simulink model "ROV_Simulator"  (R2023b)
settings: Solver=ode45  StartTime=0.0  StopTime=100  FixedStep=0.0001  MaxStep=0.0001  RelTol=1e-3
InitFcn:
  | init_params
  | 
  | vehicle_parameters_vita1_simu2vita
model workspace (MAT data in the model file):
  PID_params = [219.545279942 3.70519601588 93.8828385991 194.811835155 6.72701520051 121.59112254 154.922739587 1.92908191949 101.939011964 1.23491492885 1.15087256702 0.897835335235 0.858804638878 3.40602843271 0.73871001899 1.02484674583 4.65741084383 0.363408187927]
  PID_pitch = [0 0 0]
  PID_roll = [0 0 0]
  PID_x = [0 0 0]
  PID_y = [0 0 0]
  PID_yaw = [0.04 0 0.18]
  PID_z = [0 0 0]
values from neighbouring files (symbols this model uses):
  actuators_tconst = ones(qty_actuators, 1)*0.1754    [vehicle_parameters_vita1_simu2vita.m]
  Dlf = -[X_u;         Y_v;         Z_w;         K_p;         M_q;         N_r]    [vehicle_parameters_vita1_simu2vita.m]
  Dqf = -[X_u_u;         Y_v_v;         Z_w_w;         K_p_p;         M_q_q;         N_r_r]    [vehicle_parameters_vita1_simu2vita.m]
  I_b = diag([I_x; I_y; I_z])    [vehicle_parameters_vita1_simu2vita.m]
  init_vehicle_linear_vel = [0 0 0]'    [init_params.m]
  init_vehicle_position = [0 0 0]'    [init_params.m]
  last_waypoint_thresh = Parameters.reference.path.last_waypoint_thresh    [init_params.m]
  m = 25    [vehicle_parameters_vita1_simu2vita.m]
  Ma = -diag([X_u_dot; Y_v_dot; Z_w_dot; K_p_dot; M_q_dot; N_r_dot])    [vehicle_parameters_vita1_simu2vita.m]
  nlinear_sf = 400    [init_params.m]
  path_ref_mask = Parameters.reference.path.reference_mask    [init_params.m]
  pos_sample_freq = 4    [init_params.m]
  qty_actuators = 8    [vehicle_parameters_vita1_simu2vita.m]
  r_b = [0; 0; -0.08]    [vehicle_parameters_vita1_simu2vita.m]
  r_g = [0; 0; 0.02]    [vehicle_parameters_vita1_simu2vita.m]
  ref_switch = 1    [init_params.m]
  ref_waypoints = Parameters.reference.path.waypoints    [init_params.m]
  rho = 1028    [vehicle_parameters_vita1_simu2vita.m]
  step_signal = Parameters.reference.stage_step_signal    [init_params.m]
  thrust_inferior = ones(qty_actuators, 1)*(-39.91)    [vehicle_parameters_vita1_simu2vita.m]
  thrust_sup = ones(qty_actuators, 1)*51.48    [vehicle_parameters_vita1_simu2vita.m]
  thruster_effectiveness_matrix = thruster_effectiveness_matrix *                               thruster_effectiveness    [vehicle_parameters_vita1_simu2vita.m]
  vol = 0.02432    [vehicle_parameters_vita1_simu2vita.m]
  waypoint_thresh = Parameters.reference.path.waypoint_thresh    [init_params.m]
libraries: slpidlib x6, sharedutil x3, aerolibutil x3, sharedtransform x2, aerolibconvert2 x1, dspswit3 x1
(part 1 of 2)
settings Model: PacingRate=0.890000  Creator=spades  LastModifiedBy=HP
settings SolverCC: ConcurrentTasks=on  AlgebraicLoopSolver=TrustRegion  AutoInsertRateTranBlk=on
settings OptimizationCC: EnhancedBackFolding=on  PassReuseOutputArgsThreshold=0  MaxStackSize=64  OptimizeBlockOrder=speed  DifferentSizesBufferReuse=on
settings DebuggingCC: ReadBeforeWriteMsg=DisableAll  WriteAfterWriteMsg=DisableAll  WriteAfterReadMsg=DisableAll  InheritedTsInSrcMsg=none  ParameterTunabilityLossMsg=error  UnconnectedLineMsg=warning
settings HardwareCC: ProdBitPerLong=64  ProdHWDeviceType=Intel->x86-64 (Linux 64)
settings ModelReferenceCC: EnableRefExpFcnMdlSchedulingChecks=on
settings SFSimCC: MATLABDynamicMemAlloc=off
settings RTWCC: GenerateReport=on  Toolchain=Catkin  LaunchReport=on
settings CodeAppCC: ForceParamTrailComments=on  OperatorAnnotations=on
settings GRTTargetCC: TargetLangStandard=C89/C90 (ANSI)

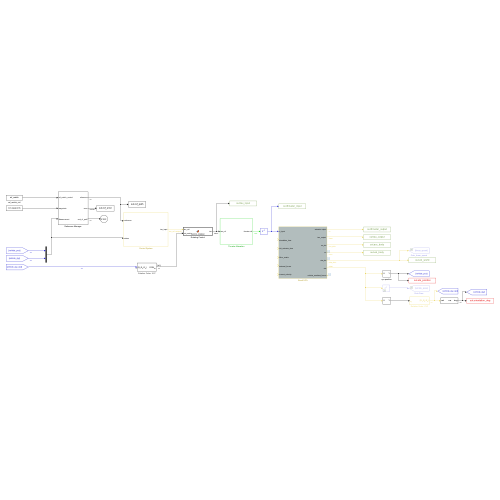
[thumbnail: Simulink's stored preview of the top-level diagram]
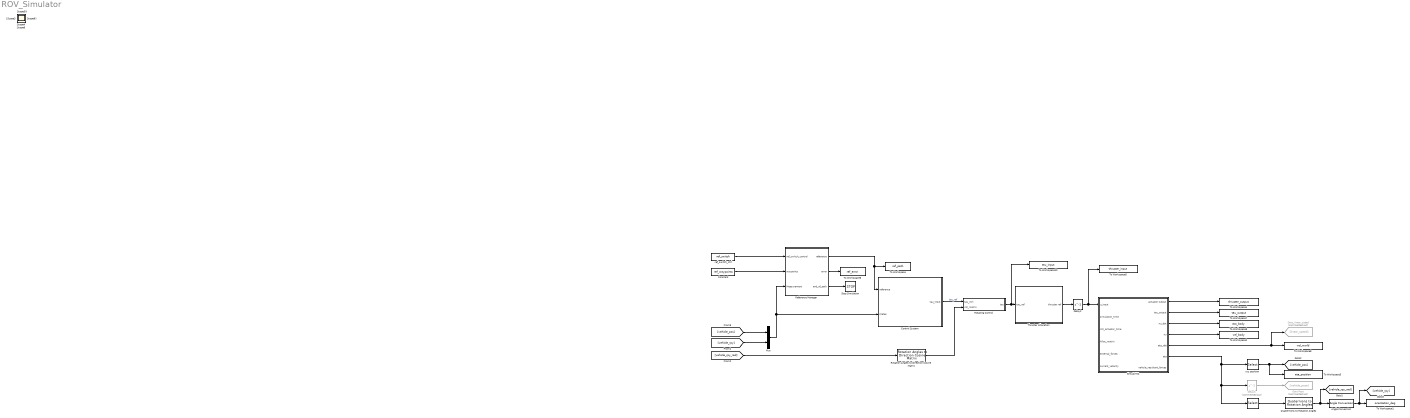
== system ROV_Simulator ==
  " " : Selector  InputPortWidth=7  IndexOptions=Index vector (dialog)  Indices=[4 5 6 7]  OutputSizes=1
  Angle Conversion : aerolibconvert2/Angle Conversion  IU=rad  OU=deg
  Constant : Constant  Value=ref_waypoints
  Control System : Subsystem
  Delay2 : Delay  DelayLength=1  InitialCondition=[0 0 0 0 0 0 0 0]'  SampleTime=1/nlinear_sf
  Delay3 : Delay  Commented=on  DelayLength=1  InitialCondition=[init_vehicle_position' init_vehicle_orientation']'  SampleTime=1/nlinear_sf
  Goto Pose : Goto  Commented=on  GotoTag=vehicle_pose
  Goto_linear_speed : Goto  Commented=on  GotoTag=linear_speed
  Mux : Mux  Inputs=2
  Quaternions to Rotation Angles : sharedtransform/Quaternions to Rotation Angles  rotationOrder=XYZ  aMode=aMode
  Reference Manager : Subsystem
  Rotating Control : MATLAB Function  TreatAsAtomicUnit=on
  Rotation Angles to Direction Cosine Matrix : sharedtransform/Rotation Angles to Direction Cosine Matrix  rotationOrder=XYZ  aMode=aMode
  Simu2VITA : Subsystem  mask{m_qty_actuators=qty_actuators, m_init_actuators_state=[0; 0; 0; 0; 0; 0; 0; 0], m_logic_op_use_custom_actuators_init_states=on, m_internal_init_actuators_time=0, m_logic_op_use_external_actuators_init_time=off, m_logic_op_use_external_time=off, m_thrust_sup=thrust_sup, m_thrust_inf=thrust_inferior, m_logic_op_thrust_saturation=on, m_actuators_tconst_vec=actuators_tconst, m_allocation_matrix=thruster_effectiveness_matrix, m_logic_op_external_alloc_mat=off, m_m=m, m_vol=vol, m_r_g=r_g, m_I_b=I_b, m_loigc_op_use_external_forces=off, m_Ma=Ma, m_Dlf_vec=Dlf, m_Dqf_vec=Dqf, m_current_velocity=[0.7 0 0]', m_loigc_op_use_external_current_velocity=off, m_g=9.81, m_rho=rho, m_r_b=r_b, m_eta_0=[init_vehicle_position' init_vehicle_orientation']', m_nu_0=[init_vehicle_linear_vel' init_vehicle_angular_vel']'}
      mask prompts: m_qty_actuators "Number of actuators on vehicle"; m_init_actuators_state "Actuators initial state values"; m_logic_op_use_custom_actuators_init_states "use custom initial state for actuators to start"; m_internal_init_actuators_time "Actuators initial time values"; m_logic_op_use_external_actuators_init_time "use custom initial time for actuators to start"; m_logic_op_use_external_time "use external clock reference"; m_thrust_sup "Thrust superior saturation limits"; m_thrust_inf "Thrust lower saturation limits"; m_logic_op_thrust_saturation "use thrust saturation"; m_actuators_tconst_vec "Time Constant values"; m_allocation_matrix "Allocation Matrix"; m_logic_op_external_alloc_mat "use external allocation matrix"; m_m "Vehicle Total Mass"; m_vol "Vehicle Total Volume"; m_r_g "Vehicle center of gravity w.r.t. vehicle control point"; m_I_b "Intertia Matrix"; m_loigc_op_use_external_forces "enable external forces and moments"; m_Ma "Addded Mass Matrix"; m_Dlf_vec "Drag Linear Factor"; m_Dqf_vec "Drag Non Linear Factor"; m_current_velocity "Fluid current velocity"; m_loigc_op_use_external_current_velocity "use external fluid current velocity"; m_g "Gravity Constant"; m_rho "Fluid Constant"; m_r_b "Vehicle center of bouyance w.r.t. vehicle body frame"; m_eta_0 "Initial pose of the vehicle -- [pos quat]'"; m_nu_0 "Initial velocity and gyros of the vehicle -- [u v w p q r]'"
      mask help: $ \eta = 0 $
      mask init:
      | assert((numel(m_qty_actuators) == 1 && m_qty_actuators >= 0), 'The number of actuators must be a non-negative   scalar.');
      | 
      | if(m_qty_actuators == 0)
      |    
      |     m_logic_op_external_alloc_mat = false;
      |     m_allocation_matrix = zeros(6,1);
      |     m_init_actuators_state = 0;
      |     m_internal_init_actuators_time = 0;
      |     m_actuators_tconst_vec = 1;
      |     m_thrust_sup = 0;
      |     m_thrust_inf = 0;
      |     m_logic_op_thrust_saturation = false;
      |     
      | else
      |     
      |     if(~m_logic_op_use_custom_actuators_init_states)
      |         m_init_actuators_state = zeros(m_qty_actuators,1);
      |     end
      |     
      |     if(~m_logic_op_use_external_actuators_init_time)
      |         m_internal_init_actuators_time = zeros(m_qty_actuators,1);
      |     end
      |     
      |     if(m_logic_op_thrust_saturation)
      |         assert(isequal(size(m_thrust_sup), [m_qty_actuators 1]));
      |         assert(isequal(size(m_thrust_inf), [m_qty_actuators 1]));
      |     end
      |     
      |     assert(isequal(size(m_init_actuators_state), [m_qty_actuators 1]), ...
      |         'Initial actuator state vector must be a column vector and agree with the number of actuators specified.');
      |     
      |     assert(isequal(size(m_internal_init_actuators_time), [m_qty_actuators 1]), ...
      |         'Initial actuator time vector must be a column vector and agree with the number of actuators specified.');
      |     
      | end
      | 
      | if(~m_logic_op_external_alloc_mat)
      | 
      |     assert(isequal(size(m_allocation_matrix), [6 numel(m_init_actuators_state)]));
      | 
      | end
      | 
      | assert(isequal(size(m_r_g), [3 1]), 'Center of gravity must be a 3x1 column vector.');
      | assert(isequal(size(m_r_b), [3 1]), 'Center of bouyancy must be a 3x1 column vector.');
      | assert(isequal(size(m_eta_0), [7 1]), 'Initial pose state w.r.t. NED must be a 7x1 column vector.');
      | assert(abs(norm(m_eta_0(4:7,1)) - 1) < 0.00001, 'Initial orientation state quaternion must have unitary norm.')
      | assert(isequal(size(m_nu_0), [6 1]), 'Initial velocity state w.r.t. body must be a 6x1 column vector.');
      | assert(isequal(size(m_I_b), [3 3]), 'Inertia matrix w.r.t. body must be a 3x3 matrix.');
      | assert(isequal(size(m_Ma), [6 6]), 'Added mass matrix must be a 6x6 matrix.');
      | assert(isequal(size(m_current_velocity), [3 1]), 'Current velocity must be a 3x1 column vector.');
      | assert(isequal(size(m_m), [1 1]), 'Mass must be a scalar.');
      | assert(isequal(size(m_vol), [1 1]), 'The volume of the vehicle must be a scalar.');
      | assert(isequal(size(m_g), [1 1]), 'Gravity must be a scalar.');
      | assert(isequal(size(m_rho), [1 1]), 'Fluid density must be a scalar.');
      | assert(isequal(size(m_Dlf_vec), [6 1]), 'Linear Drag Matrix is assumed to be diagonal and should be entered as a 6x1 vector.');
      | assert(isequal(size(m_Dqf_vec), [6 1]), 'Non-Linear Drag Matrix is assumed to be diagonal and should be entered as a 6x1 vector.');
      | 
      | m_W = m_m*m_g;
      | 
      | m_B = -m_vol*m_g*m_rho;
      | 
      | m_Smtrx_r_g = [0 -m_r_g(3) m_r_g(2); ... 
      |              m_r_g(3) 0 -m_r_g(1); ... 
      |             -m_r_g(2) m_r_g(1) 0];  
      | 
      | m_M = [m_m*eye(3) -m_m*m_Smtrx_r_g; ...
      |      m_m*m_Smtrx_r_g m_I_b];
      | 
      | m_Dlf = diag(m_Dlf_vec);
      | m_Dqf = diag(m_Dqf_vec);
      | 
      | m_Ad = diag((-1./m_actuators_tconst_vec));
      | m_Bd = -m_Ad;
      | m_Cd = diag(ones(size(m_Ad, 2), 1));
      | m_Dd = zeros(numel(m_actuators_tconst_vec), numel(m_actuators_tconst_vec));
      mask Callback m_logic_op_use_custom_actuators_init_states:
      | p = Simulink.Mask.get(gcb);
      | a = p.Parameters(2);
      | 
      | cur_param_val_on = ...
      |     (strcmp(get_param(gcb, 'm_logic_op_use_custom_actuators_init_states'), 'on') ~= 0);
      | 
      | if (cur_param_val_on)
      | 
      |     for i = 1
      |         a(i).set('Enabled', 'on');
      |     end
      | 
      | else
      | 
      |     for i = 1
      |         a(i).set('Enabled', 'off');
      |     end
      | 
      | end
      mask Callback m_logic_op_use_external_actuators_init_time:
      | p = Simulink.Mask.get(gcb);
      | a = p.Parameters(4);
      | 
      | cur_param_val_on = ...
      |     (strcmp(get_param(gcb, 'm_logic_op_use_external_actuators_init_time'), 'on') ~= 0);
      | 
      | if (cur_param_val_on)
      | 
      |     for i = 1
      |         a(i).set('Enabled', 'on');
      |     end
      | 
      | else
      | 
      |     for i = 1
      |         a(i).set('Enabled', 'off');
      |     end
      | 
      | end
      mask Callback m_logic_op_thrust_saturation:
      | p = Simulink.Mask.get(gcb);
      | a = p.Parameters(7:8);
      | 
      | cur_param_val_on = ...
      |     (strcmp(get_param(gcb, 'm_logic_op_thrust_saturation'), 'on') ~= 0);
      | 
      | if (cur_param_val_on)
      | 
      |     for i = 1:2
      |         a(i).set('Enabled', 'on');
      |     end
      | 
      | else
      | 
      |     for i = 1:2
      |         a(i).set('Enabled', 'off');
      |     end
      | 
      | end
      mask Callback m_logic_op_external_alloc_mat:
      | p = Simulink.Mask.get(gcb);
      | a = p.Parameters(11);
      | 
      | cur_param_val_on = ...
      |     (strcmp(get_param(gcb, 'm_logic_op_external_alloc_mat'), 'on') ~= 0);
      | 
      | if (cur_param_val_on)
      | 
      |     for i = 1
      |         a(i).set('Enabled', 'off');
      |     end
      | 
      | else
      | 
      |     for i = 1
      |         a(i).set('Enabled', 'on');
      |     end
      | 
      | end
      mask Callback m_loigc_op_use_external_current_velocity:
      | p = Simulink.Mask.get(gcb);
      | a = p.Parameters(21);
      | 
      | cur_param_val_on = ...
      |     (strcmp(get_param(gcb, 'm_loigc_op_use_external_current_velocity'), 'on') ~= 0);
      | 
      | if (cur_param_val_on)
      | 
      |     for i = 1
      |         a(i).set('Enabled', 'off');
      |     end
      | 
      | else
      | 
      |     for i = 1
      |         a(i).set('Enabled', 'on');
      |     end
      | 
      | end
      mask DialogControl act_system Prompt: Actuator Module
      mask DialogControl act_start_group Prompt: Start options
      mask DialogControl thrust_sat_options Prompt: Thrust saturation options
      mask DialogControl act_evo_group Prompt: Evolution options
      mask DialogControl vehicle_input_tab Prompt: Allocation Module
      mask DialogControl vehicle_dynamic_tab Prompt: Vehicle Dynamic Parameters
      mask DialogControl rigid_body_comp Prompt: Rigid-body Components
      mask DialogControl m_vol Tooltip: Liters
      mask DialogControl hydro_dynam_comp Prompt: Hydrodanymic Components
      mask DialogControl hydro_static_comp Prompt: Hydrostatic Components
      mask DialogControl init_state Prompt: Initial state of the vehicle
      mask DialogControl m_eta_0 Tooltip: Pose state of the vehicle [pose quat]', with pose in meters w.r.t. NED
  Stop Simulation : Stop
  Thruster Allocation : Subsystem
  To Workspace : ToWorkspace  VariableName=ref_path  SaveFormat=Timeseries  SampleTime=-1
  To Workspace1 : ToWorkspace  VariableName=orientation_deg  SaveFormat=Timeseries  SampleTime=-1
  To Workspace10 : ToWorkspace  VariableName=tau_input  SaveFormat=Timeseries  SampleTime=-1
  To Workspace2 : ToWorkspace  VariableName=vel_body  SaveFormat=Timeseries  SampleTime=1/pos_sample_freq
  To Workspace3 : ToWorkspace  VariableName=eta_position  SaveFormat=Timeseries  SampleTime=-1
  To Workspace4 : ToWorkspace  VariableName=thruster_output  SaveFormat=Timeseries  SampleTime=-1
  To Workspace5 : ToWorkspace  VariableName=thruster_input  SaveFormat=Timeseries  SampleTime=-1
  To Workspace6 : ToWorkspace  VariableName=ref_error  SaveFormat=Timeseries  SampleTime=-1
  To Workspace7 : ToWorkspace  VariableName=tau_output  SaveFormat=Timeseries  SampleTime=-1
  To Workspace8 : ToWorkspace  VariableName=vel_world  SaveFormat=Timeseries  SampleTime=1/pos_sample_freq
  To Workspace9 : ToWorkspace  VariableName=acc_body  SaveFormat=Timeseries  SampleTime=1/pos_sample_freq
  ref_switch_ctrl : Constant  Value=ref_switch
  xyz position : Selector  InputPortWidth=7  IndexOptions=Index vector (dialog)  Indices=[1 2 3]  OutputSizes=1
  Scope{,1..6,9..10,13..15,18..19} (14 alike) : Scope
  wires:
  Simu2VITA/6(eta) -> " "/1, Delay3/1, xyz position/1
  Delay3/1 -> Goto Pose/1
  Simu2VITA/4(nu) -> To Workspace2/1
  xyz position/1 -> [vehicle_pos], To Workspace3/1
  " "/1 -> Quaternions to Rotation Angles/1
  Quaternions to Rotation Angles/1 -> Angle Conversion/1, [vehicle_rpy_rad]
  Simu2VITA/1(actuator output) -> To Workspace4/1
  Simu2VITA/5(eta_dot) -> To Workspace8/1, Goto_linear_speed/1
  [vehicle_pos] -> Mux/1
  Mux/1 -> Reference Manager/3(Measurement), Control System/2(states)
  [vehicle_rpy] -> Mux/2
  Simu2VITA/2("tau_output ") -> To Workspace7/1
  Simu2VITA/3(nu_dot) -> To Workspace9/1
  Thruster Allocation/1(thruster ref) -> Delay2/1
  Delay2/1 -> To Workspace5/1, Simu2VITA/1(u_input)
  Rotation Angles to Direction Cosine Matrix/1 -> Rotating Control/2(rot_matrix)
  [vehicle_rpy_rad] -> Rotation Angles to Direction Cosine Matrix/1
  Control System/1(tau_input) -> Rotating Control/1(tau_ctrl)  "tau_ref"
  Angle Conversion/1 -> [vehicle_rpy], To Workspace1/1
  Rotating Control/1(tau) -> To Workspace10/1, Thruster Allocation/1(tau_ref)
  Reference Manager/1(reference) -> To Workspace/1, Control System/1(reference)
  Reference Manager/2(error) -> To Workspace6/1
  ref_switch_ctrl/1 -> Reference Manager/1(ref_switch_control)
  Constant/1 -> Reference Manager/2(waypoints)
  Reference Manager/3(end_of_path) -> Stop Simulation/1

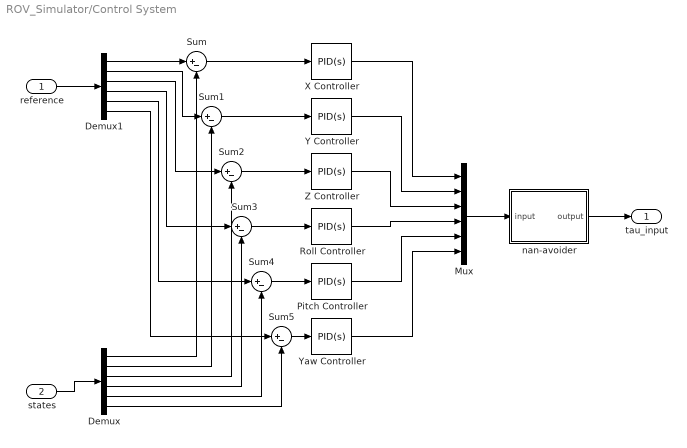
== system ROV_Simulator/Control System ==
  reference : Inport
  states : Inport  Port=2
  Demux : Demux  Outputs=6
  Demux1 : Demux  Outputs=6
  Mux : Mux  Inputs=6
  Pitch Controller : slpidlib/PID Controller  Controller=PID  Form=Parallel  TimeDomain=Continuous-time  UseExternalTs=off  SampleTime=-1  IntegratorMethod=Forward Euler  FilterMethod=Forward Euler  ControllerParametersSource=internal  P=PID_params(13)  I=PID_params(14)  UseKiTs=off  D=PID_params(15)  N=100  UseFilter=on  TunerSelectOption=Transfer Function Based (PID Tuner App)  InitialConditionSource=internal  InitialConditionForIntegrator=0  InitialConditionForFilter=0  DifferentiatorICPrevScaledInput=0  ExternalReset=none  TrackingMode=off  Kt=1  LimitOutput=off  SatLimitsSource=internal  UpperSaturationLimit=inf  LowerSaturationLimit=-inf  LinearizeAsGain=on  AntiWindupMode=none  Kb=1  LimitIntegrator=off  UpperIntegratorSaturationLimit=inf  LowerIntegratorSaturationLimit=-inf  POutMin=[]  POutMax=[]  IOutMin=[]  IOutMax=[]  DOutMin=[]  DOutMax=[]  NOutMin=[]  NOutMax=[]  SumOutMin=[]  SumOutMax=[]  SaturationOutMin=[]  SaturationOutMax=[]  PParamMin=[]  PParamMax=[]  IParamMin=[]  IParamMax=[]  DParamMin=[]  DParamMax=[]  NParamMin=[]  NParamMax=[]  KbParamMin=[]  KbParamMax=[]  KtParamMin=[]  KtParamMax=[]  KbOutMin=[]  KbOutMax=[]  KtOutMin=[]  KtOutMax=[]  IntegratorOutMin=[]  IntegratorOutMax=[]  FilterOutMin=[]  FilterOutMax=[]  SumI1OutMin=[]  SumI1OutMax=[]  SumI2OutMin=[]  SumI2OutMax=[]  SumI3OutMin=[]  SumI3OutMax=[]  SumI4OutMin=[]  SumI4OutMax=[]  SumDOutMin=[]  SumDOutMax=[]  DifferentiatorOutMin=[]  DifferentiatorOutMax=[]  FilterDiffOutCoefMin=[]  FilterDiffOutCoefMax=[]  ReciprocalOutMin=[]  ReciprocalOutMax=[]  SumDenOutMin=[]  SumDenOutMax=[]  SumNumOutMin=[]  SumNumOutMax=[]  DivideOutMin=[]  DivideOutMax=[]  UdiffTsProdOutMin=[]  UdiffTsProdOutMax=[]  NTsProdOutMin=[]  NTsProdOutMax=[]  UintegralTsProdOutMin=[]  UintegralTsProdOutMax=[]  UngainTsProdOutMin=[]  UngainTsProdOutMax=[]  ClampingZeroOutDataTypeStr=Inherit: Inherit via back propagation  ClampingZeroOutMin=[]  ClampingZeroOutMax=[]  FilterDenConstantOutDataTypeStr=Inherit: Inherit via back propagation  FilterDenConstantOutMin=[]  FilterDenConstantOutMax=[]  PCopyOutDataTypeStr=Inherit: Inherit via back propagation  PCopyOutMin=[]  PCopyOutMax=[]  NCopyOutDataTypeStr=Inherit: Inherit via back propagation  NCopyOutMin=[]  NCopyOutMax=[]  IntegratorContinuousStateAttributes=''  IntegratorStateMustResolveToSignalObject=off  IntegratorRTWStateStorageClass=Auto  FilterContinuousStateAttributes=''  FilterStateMustResolveToSignalObject=off  FilterRTWStateStorageClass=Auto  ParallelPVariant=InternalParameters  IdealPVariant=Disabled  IVariant=InternalParameters  DVariant=InternalParameters  IntegratorVariant=Continuous  SatVariant=Disabled  AWVariant=Passthrough  PCopyVariant=Disabled  TRVariant=Disabled  FdbkBlocksVariant=Forward  IdealPFdbkVariant=Disabled  SatFdbkVariant=Disabled  DerivativeFilterVariant=ContFilter  NVariant=InternalParameters  NCopyVariant=Disabled  FilterICVariant=InternalICsFilter  IntegratorICVariant=InternalICs  ExternalResetVariant=Disabled  TRSumVariant=Passthrough  SumFdbkVariant=Disabled  SumVariant=Sum_PID  TsampFilterVariant=InternalTs  TsampNgainVariant=Passthrough  TsampIntegralVariant=Disabled_SignalSpec  ExternalSaturationOutDataTypeStr=Inherit: Same as second input
  Roll Controller : slpidlib/PID Controller  Controller=PID  Form=Parallel  TimeDomain=Continuous-time  UseExternalTs=off  SampleTime=-1  IntegratorMethod=Forward Euler  FilterMethod=Forward Euler  ControllerParametersSource=internal  P=PID_params(10)  I=PID_params(11)  UseKiTs=off  D=PID_params(12)  N=100  UseFilter=on  TunerSelectOption=Transfer Function Based (PID Tuner App)  InitialConditionSource=internal  InitialConditionForIntegrator=0  InitialConditionForFilter=0  DifferentiatorICPrevScaledInput=0  ExternalReset=none  TrackingMode=off  Kt=1  LimitOutput=off  SatLimitsSource=internal  UpperSaturationLimit=inf  LowerSaturationLimit=-inf  LinearizeAsGain=on  AntiWindupMode=none  Kb=1  LimitIntegrator=off  UpperIntegratorSaturationLimit=inf  LowerIntegratorSaturationLimit=-inf  POutMin=[]  POutMax=[]  IOutMin=[]  IOutMax=[]  DOutMin=[]  DOutMax=[]  NOutMin=[]  NOutMax=[]  SumOutMin=[]  SumOutMax=[]  SaturationOutMin=[]  SaturationOutMax=[]  PParamMin=[]  PParamMax=[]  IParamMin=[]  IParamMax=[]  DParamMin=[]  DParamMax=[]  NParamMin=[]  NParamMax=[]  KbParamMin=[]  KbParamMax=[]  KtParamMin=[]  KtParamMax=[]  KbOutMin=[]  KbOutMax=[]  KtOutMin=[]  KtOutMax=[]  IntegratorOutMin=[]  IntegratorOutMax=[]  FilterOutMin=[]  FilterOutMax=[]  SumI1OutMin=[]  SumI1OutMax=[]  SumI2OutMin=[]  SumI2OutMax=[]  SumI3OutMin=[]  SumI3OutMax=[]  SumI4OutMin=[]  SumI4OutMax=[]  SumDOutMin=[]  SumDOutMax=[]  DifferentiatorOutMin=[]  DifferentiatorOutMax=[]  FilterDiffOutCoefMin=[]  FilterDiffOutCoefMax=[]  ReciprocalOutMin=[]  ReciprocalOutMax=[]  SumDenOutMin=[]  SumDenOutMax=[]  SumNumOutMin=[]  SumNumOutMax=[]  DivideOutMin=[]  DivideOutMax=[]  UdiffTsProdOutMin=[]  UdiffTsProdOutMax=[]  NTsProdOutMin=[]  NTsProdOutMax=[]  UintegralTsProdOutMin=[]  UintegralTsProdOutMax=[]  UngainTsProdOutMin=[]  UngainTsProdOutMax=[]  ClampingZeroOutDataTypeStr=Inherit: Inherit via back propagation  ClampingZeroOutMin=[]  ClampingZeroOutMax=[]  FilterDenConstantOutDataTypeStr=Inherit: Inherit via back propagation  FilterDenConstantOutMin=[]  FilterDenConstantOutMax=[]  PCopyOutDataTypeStr=Inherit: Inherit via back propagation  PCopyOutMin=[]  PCopyOutMax=[]  NCopyOutDataTypeStr=Inherit: Inherit via back propagation  NCopyOutMin=[]  NCopyOutMax=[]  IntegratorContinuousStateAttributes=''  IntegratorStateMustResolveToSignalObject=off  IntegratorRTWStateStorageClass=Auto  FilterContinuousStateAttributes=''  FilterStateMustResolveToSignalObject=off  FilterRTWStateStorageClass=Auto  ParallelPVariant=InternalParameters  IdealPVariant=Disabled  IVariant=InternalParameters  DVariant=InternalParameters  IntegratorVariant=Continuous  SatVariant=Disabled  AWVariant=Passthrough  PCopyVariant=Disabled  TRVariant=Disabled  FdbkBlocksVariant=Forward  IdealPFdbkVariant=Disabled  SatFdbkVariant=Disabled  DerivativeFilterVariant=ContFilter  NVariant=InternalParameters  NCopyVariant=Disabled  FilterICVariant=InternalICsFilter  IntegratorICVariant=InternalICs  ExternalResetVariant=Disabled  TRSumVariant=Passthrough  SumFdbkVariant=Disabled  SumVariant=Sum_PID  TsampFilterVariant=InternalTs  TsampNgainVariant=Passthrough  TsampIntegralVariant=Disabled_SignalSpec  ExternalSaturationOutDataTypeStr=Inherit: Same as second input
  Sum{,1..5} (6 alike) : Sum  Inputs=|+-
  X Controller : slpidlib/PID Controller  Controller=PID  Form=Parallel  TimeDomain=Continuous-time  UseExternalTs=off  SampleTime=-1  IntegratorMethod=Forward Euler  FilterMethod=Forward Euler  ControllerParametersSource=internal  P=PID_params(1)  I=PID_params(2)  UseKiTs=off  D=PID_params(3)  N=100  UseFilter=on  TunerSelectOption=Transfer Function Based (PID Tuner App)  InitialConditionSource=internal  InitialConditionForIntegrator=0  InitialConditionForFilter=0  DifferentiatorICPrevScaledInput=0  ExternalReset=none  TrackingMode=off  Kt=1  LimitOutput=off  SatLimitsSource=internal  UpperSaturationLimit=inf  LowerSaturationLimit=-inf  LinearizeAsGain=on  AntiWindupMode=none  Kb=1  LimitIntegrator=off  UpperIntegratorSaturationLimit=inf  LowerIntegratorSaturationLimit=-inf  POutMin=[]  POutMax=[]  IOutMin=[]  IOutMax=[]  DOutMin=[]  DOutMax=[]  NOutMin=[]  NOutMax=[]  SumOutMin=[]  SumOutMax=[]  SaturationOutMin=[]  SaturationOutMax=[]  PParamMin=[]  PParamMax=[]  IParamMin=[]  IParamMax=[]  DParamMin=[]  DParamMax=[]  NParamMin=[]  NParamMax=[]  KbParamMin=[]  KbParamMax=[]  KtParamMin=[]  KtParamMax=[]  KbOutMin=[]  KbOutMax=[]  KtOutMin=[]  KtOutMax=[]  IntegratorOutMin=[]  IntegratorOutMax=[]  FilterOutMin=[]  FilterOutMax=[]  SumI1OutMin=[]  SumI1OutMax=[]  SumI2OutMin=[]  SumI2OutMax=[]  SumI3OutMin=[]  SumI3OutMax=[]  SumI4OutMin=[]  SumI4OutMax=[]  SumDOutMin=[]  SumDOutMax=[]  DifferentiatorOutMin=[]  DifferentiatorOutMax=[]  FilterDiffOutCoefMin=[]  FilterDiffOutCoefMax=[]  ReciprocalOutMin=[]  ReciprocalOutMax=[]  SumDenOutMin=[]  SumDenOutMax=[]  SumNumOutMin=[]  SumNumOutMax=[]  DivideOutMin=[]  DivideOutMax=[]  UdiffTsProdOutMin=[]  UdiffTsProdOutMax=[]  NTsProdOutMin=[]  NTsProdOutMax=[]  UintegralTsProdOutMin=[]  UintegralTsProdOutMax=[]  UngainTsProdOutMin=[]  UngainTsProdOutMax=[]  ClampingZeroOutDataTypeStr=Inherit: Inherit via back propagation  ClampingZeroOutMin=[]  ClampingZeroOutMax=[]  FilterDenConstantOutDataTypeStr=Inherit: Inherit via back propagation  FilterDenConstantOutMin=[]  FilterDenConstantOutMax=[]  PCopyOutDataTypeStr=Inherit: Inherit via back propagation  PCopyOutMin=[]  PCopyOutMax=[]  NCopyOutDataTypeStr=Inherit: Inherit via back propagation  NCopyOutMin=[]  NCopyOutMax=[]  IntegratorContinuousStateAttributes=''  IntegratorStateMustResolveToSignalObject=off  IntegratorRTWStateStorageClass=Auto  FilterContinuousStateAttributes=''  FilterStateMustResolveToSignalObject=off  FilterRTWStateStorageClass=Auto  ParallelPVariant=InternalParameters  IdealPVariant=Disabled  IVariant=InternalParameters  DVariant=InternalParameters  IntegratorVariant=Continuous  SatVariant=Disabled  AWVariant=Passthrough  PCopyVariant=Disabled  TRVariant=Disabled  FdbkBlocksVariant=Forward  IdealPFdbkVariant=Disabled  SatFdbkVariant=Disabled  DerivativeFilterVariant=ContFilter  NVariant=InternalParameters  NCopyVariant=Disabled  FilterICVariant=InternalICsFilter  IntegratorICVariant=InternalICs  ExternalResetVariant=Disabled  TRSumVariant=Passthrough  SumFdbkVariant=Disabled  SumVariant=Sum_PID  TsampFilterVariant=InternalTs  TsampNgainVariant=Passthrough  TsampIntegralVariant=Disabled_SignalSpec  ExternalSaturationOutDataTypeStr=Inherit: Same as second input
  Y Controller : slpidlib/PID Controller  Controller=PID  Form=Parallel  TimeDomain=Continuous-time  UseExternalTs=off  SampleTime=-1  IntegratorMethod=Forward Euler  FilterMethod=Forward Euler  ControllerParametersSource=internal  P=PID_params(4)  I=PID_params(5)  UseKiTs=off  D=PID_params(6)  N=100  UseFilter=on  TunerSelectOption=Transfer Function Based (PID Tuner App)  InitialConditionSource=internal  InitialConditionForIntegrator=0  InitialConditionForFilter=0  DifferentiatorICPrevScaledInput=0  ExternalReset=none  TrackingMode=off  Kt=1  LimitOutput=off  SatLimitsSource=internal  UpperSaturationLimit=inf  LowerSaturationLimit=-inf  LinearizeAsGain=on  AntiWindupMode=none  Kb=1  LimitIntegrator=off  UpperIntegratorSaturationLimit=inf  LowerIntegratorSaturationLimit=-inf  POutMin=[]  POutMax=[]  IOutMin=[]  IOutMax=[]  DOutMin=[]  DOutMax=[]  NOutMin=[]  NOutMax=[]  SumOutMin=[]  SumOutMax=[]  SaturationOutMin=[]  SaturationOutMax=[]  PParamMin=[]  PParamMax=[]  IParamMin=[]  IParamMax=[]  DParamMin=[]  DParamMax=[]  NParamMin=[]  NParamMax=[]  KbParamMin=[]  KbParamMax=[]  KtParamMin=[]  KtParamMax=[]  KbOutMin=[]  KbOutMax=[]  KtOutMin=[]  KtOutMax=[]  IntegratorOutMin=[]  IntegratorOutMax=[]  FilterOutMin=[]  FilterOutMax=[]  SumI1OutMin=[]  SumI1OutMax=[]  SumI2OutMin=[]  SumI2OutMax=[]  SumI3OutMin=[]  SumI3OutMax=[]  SumI4OutMin=[]  SumI4OutMax=[]  SumDOutMin=[]  SumDOutMax=[]  DifferentiatorOutMin=[]  DifferentiatorOutMax=[]  FilterDiffOutCoefMin=[]  FilterDiffOutCoefMax=[]  ReciprocalOutMin=[]  ReciprocalOutMax=[]  SumDenOutMin=[]  SumDenOutMax=[]  SumNumOutMin=[]  SumNumOutMax=[]  DivideOutMin=[]  DivideOutMax=[]  UdiffTsProdOutMin=[]  UdiffTsProdOutMax=[]  NTsProdOutMin=[]  NTsProdOutMax=[]  UintegralTsProdOutMin=[]  UintegralTsProdOutMax=[]  UngainTsProdOutMin=[]  UngainTsProdOutMax=[]  ClampingZeroOutDataTypeStr=Inherit: Inherit via back propagation  ClampingZeroOutMin=[]  ClampingZeroOutMax=[]  FilterDenConstantOutDataTypeStr=Inherit: Inherit via back propagation  FilterDenConstantOutMin=[]  FilterDenConstantOutMax=[]  PCopyOutDataTypeStr=Inherit: Inherit via back propagation  PCopyOutMin=[]  PCopyOutMax=[]  NCopyOutDataTypeStr=Inherit: Inherit via back propagation  NCopyOutMin=[]  NCopyOutMax=[]  IntegratorContinuousStateAttributes=''  IntegratorStateMustResolveToSignalObject=off  IntegratorRTWStateStorageClass=Auto  FilterContinuousStateAttributes=''  FilterStateMustResolveToSignalObject=off  FilterRTWStateStorageClass=Auto  ParallelPVariant=InternalParameters  IdealPVariant=Disabled  IVariant=InternalParameters  DVariant=InternalParameters  IntegratorVariant=Continuous  SatVariant=Disabled  AWVariant=Passthrough  PCopyVariant=Disabled  TRVariant=Disabled  FdbkBlocksVariant=Forward  IdealPFdbkVariant=Disabled  SatFdbkVariant=Disabled  DerivativeFilterVariant=ContFilter  NVariant=InternalParameters  NCopyVariant=Disabled  FilterICVariant=InternalICsFilter  IntegratorICVariant=InternalICs  ExternalResetVariant=Disabled  TRSumVariant=Passthrough  SumFdbkVariant=Disabled  SumVariant=Sum_PID  TsampFilterVariant=InternalTs  TsampNgainVariant=Passthrough  TsampIntegralVariant=Disabled_SignalSpec  ExternalSaturationOutDataTypeStr=Inherit: Same as second input
  Yaw Controller : slpidlib/PID Controller  Controller=PID  Form=Parallel  TimeDomain=Continuous-time  UseExternalTs=off  SampleTime=-1  IntegratorMethod=Forward Euler  FilterMethod=Forward Euler  ControllerParametersSource=internal  P=PID_params(16)  I=PID_params(17)  UseKiTs=off  D=PID_params(18)  N=100  UseFilter=on  TunerSelectOption=Transfer Function Based (PID Tuner App)  InitialConditionSource=internal  InitialConditionForIntegrator=0  InitialConditionForFilter=0  DifferentiatorICPrevScaledInput=0  ExternalReset=none  TrackingMode=off  Kt=1  LimitOutput=off  SatLimitsSource=internal  UpperSaturationLimit=inf  LowerSaturationLimit=-inf  LinearizeAsGain=on  AntiWindupMode=none  Kb=1  LimitIntegrator=off  UpperIntegratorSaturationLimit=inf  LowerIntegratorSaturationLimit=-inf  POutMin=[]  POutMax=[]  IOutMin=[]  IOutMax=[]  DOutMin=[]  DOutMax=[]  NOutMin=[]  NOutMax=[]  SumOutMin=[]  SumOutMax=[]  SaturationOutMin=[]  SaturationOutMax=[]  PParamMin=[]  PParamMax=[]  IParamMin=[]  IParamMax=[]  DParamMin=[]  DParamMax=[]  NParamMin=[]  NParamMax=[]  KbParamMin=[]  KbParamMax=[]  KtParamMin=[]  KtParamMax=[]  KbOutMin=[]  KbOutMax=[]  KtOutMin=[]  KtOutMax=[]  IntegratorOutMin=[]  IntegratorOutMax=[]  FilterOutMin=[]  FilterOutMax=[]  SumI1OutMin=[]  SumI1OutMax=[]  SumI2OutMin=[]  SumI2OutMax=[]  SumI3OutMin=[]  SumI3OutMax=[]  SumI4OutMin=[]  SumI4OutMax=[]  SumDOutMin=[]  SumDOutMax=[]  DifferentiatorOutMin=[]  DifferentiatorOutMax=[]  FilterDiffOutCoefMin=[]  FilterDiffOutCoefMax=[]  ReciprocalOutMin=[]  ReciprocalOutMax=[]  SumDenOutMin=[]  SumDenOutMax=[]  SumNumOutMin=[]  SumNumOutMax=[]  DivideOutMin=[]  DivideOutMax=[]  UdiffTsProdOutMin=[]  UdiffTsProdOutMax=[]  NTsProdOutMin=[]  NTsProdOutMax=[]  UintegralTsProdOutMin=[]  UintegralTsProdOutMax=[]  UngainTsProdOutMin=[]  UngainTsProdOutMax=[]  ClampingZeroOutDataTypeStr=Inherit: Inherit via back propagation  ClampingZeroOutMin=[]  ClampingZeroOutMax=[]  FilterDenConstantOutDataTypeStr=Inherit: Inherit via back propagation  FilterDenConstantOutMin=[]  FilterDenConstantOutMax=[]  PCopyOutDataTypeStr=Inherit: Inherit via back propagation  PCopyOutMin=[]  PCopyOutMax=[]  NCopyOutDataTypeStr=Inherit: Inherit via back propagation  NCopyOutMin=[]  NCopyOutMax=[]  IntegratorContinuousStateAttributes=''  IntegratorStateMustResolveToSignalObject=off  IntegratorRTWStateStorageClass=Auto  FilterContinuousStateAttributes=''  FilterStateMustResolveToSignalObject=off  FilterRTWStateStorageClass=Auto  ParallelPVariant=InternalParameters  IdealPVariant=Disabled  IVariant=InternalParameters  DVariant=InternalParameters  IntegratorVariant=Continuous  SatVariant=Disabled  AWVariant=Passthrough  PCopyVariant=Disabled  TRVariant=Disabled  FdbkBlocksVariant=Forward  IdealPFdbkVariant=Disabled  SatFdbkVariant=Disabled  DerivativeFilterVariant=ContFilter  NVariant=InternalParameters  NCopyVariant=Disabled  FilterICVariant=InternalICsFilter  IntegratorICVariant=InternalICs  ExternalResetVariant=Disabled  TRSumVariant=Passthrough  SumFdbkVariant=Disabled  SumVariant=Sum_PID  TsampFilterVariant=InternalTs  TsampNgainVariant=Passthrough  TsampIntegralVariant=Disabled_SignalSpec  ExternalSaturationOutDataTypeStr=Inherit: Same as second input
  Z Controller : slpidlib/PID Controller  Controller=PID  Form=Parallel  TimeDomain=Continuous-time  UseExternalTs=off  SampleTime=-1  IntegratorMethod=Forward Euler  FilterMethod=Forward Euler  ControllerParametersSource=internal  P=PID_params(7)  I=PID_params(8)  UseKiTs=off  D=PID_params(9)  N=100  UseFilter=on  TunerSelectOption=Transfer Function Based (PID Tuner App)  InitialConditionSource=internal  InitialConditionForIntegrator=0  InitialConditionForFilter=0  DifferentiatorICPrevScaledInput=0  ExternalReset=none  TrackingMode=off  Kt=1  LimitOutput=off  SatLimitsSource=internal  UpperSaturationLimit=inf  LowerSaturationLimit=-inf  LinearizeAsGain=on  AntiWindupMode=none  Kb=1  LimitIntegrator=off  UpperIntegratorSaturationLimit=inf  LowerIntegratorSaturationLimit=-inf  POutMin=[]  POutMax=[]  IOutMin=[]  IOutMax=[]  DOutMin=[]  DOutMax=[]  NOutMin=[]  NOutMax=[]  SumOutMin=[]  SumOutMax=[]  SaturationOutMin=[]  SaturationOutMax=[]  PParamMin=[]  PParamMax=[]  IParamMin=[]  IParamMax=[]  DParamMin=[]  DParamMax=[]  NParamMin=[]  NParamMax=[]  KbParamMin=[]  KbParamMax=[]  KtParamMin=[]  KtParamMax=[]  KbOutMin=[]  KbOutMax=[]  KtOutMin=[]  KtOutMax=[]  IntegratorOutMin=[]  IntegratorOutMax=[]  FilterOutMin=[]  FilterOutMax=[]  SumI1OutMin=[]  SumI1OutMax=[]  SumI2OutMin=[]  SumI2OutMax=[]  SumI3OutMin=[]  SumI3OutMax=[]  SumI4OutMin=[]  SumI4OutMax=[]  SumDOutMin=[]  SumDOutMax=[]  DifferentiatorOutMin=[]  DifferentiatorOutMax=[]  FilterDiffOutCoefMin=[]  FilterDiffOutCoefMax=[]  ReciprocalOutMin=[]  ReciprocalOutMax=[]  SumDenOutMin=[]  SumDenOutMax=[]  SumNumOutMin=[]  SumNumOutMax=[]  DivideOutMin=[]  DivideOutMax=[]  UdiffTsProdOutMin=[]  UdiffTsProdOutMax=[]  NTsProdOutMin=[]  NTsProdOutMax=[]  UintegralTsProdOutMin=[]  UintegralTsProdOutMax=[]  UngainTsProdOutMin=[]  UngainTsProdOutMax=[]  ClampingZeroOutDataTypeStr=Inherit: Inherit via back propagation  ClampingZeroOutMin=[]  ClampingZeroOutMax=[]  FilterDenConstantOutDataTypeStr=Inherit: Inherit via back propagation  FilterDenConstantOutMin=[]  FilterDenConstantOutMax=[]  PCopyOutDataTypeStr=Inherit: Inherit via back propagation  PCopyOutMin=[]  PCopyOutMax=[]  NCopyOutDataTypeStr=Inherit: Inherit via back propagation  NCopyOutMin=[]  NCopyOutMax=[]  IntegratorContinuousStateAttributes=''  IntegratorStateMustResolveToSignalObject=off  IntegratorRTWStateStorageClass=Auto  FilterContinuousStateAttributes=''  FilterStateMustResolveToSignalObject=off  FilterRTWStateStorageClass=Auto  ParallelPVariant=InternalParameters  IdealPVariant=Disabled  IVariant=InternalParameters  DVariant=InternalParameters  IntegratorVariant=Continuous  SatVariant=Disabled  AWVariant=Passthrough  PCopyVariant=Disabled  TRVariant=Disabled  FdbkBlocksVariant=Forward  IdealPFdbkVariant=Disabled  SatFdbkVariant=Disabled  DerivativeFilterVariant=ContFilter  NVariant=InternalParameters  NCopyVariant=Disabled  FilterICVariant=InternalICsFilter  IntegratorICVariant=InternalICs  ExternalResetVariant=Disabled  TRSumVariant=Passthrough  SumFdbkVariant=Disabled  SumVariant=Sum_PID  TsampFilterVariant=InternalTs  TsampNgainVariant=Passthrough  TsampIntegralVariant=Disabled_SignalSpec  ExternalSaturationOutDataTypeStr=Inherit: Same as second input
  nan-avoider : MATLAB Function
  tau_input : Outport  VectorParamsAs1DForOutWhenUnconnected=off
  wires:
  Mux/1 -> nan-avoider/1(input)
  nan-avoider/1(output) -> tau_input/1
  Sum/1 -> X Controller/1
  Sum1/1 -> Y Controller/1
  Sum2/1 -> Z Controller/1
  Sum3/1 -> Roll Controller/1
  Sum4/1 -> Pitch Controller/1
  Sum5/1 -> Yaw Controller/1
  X Controller/1 -> Mux/1
  Y Controller/1 -> Mux/2
  Z Controller/1 -> Mux/3
  Roll Controller/1 -> Mux/4
  Pitch Controller/1 -> Mux/5
  Yaw Controller/1 -> Mux/6
  states/1 -> Demux/1
  Demux/1 -> Sum/2
  Demux/2 -> Sum1/2
  Demux/3 -> Sum2/2
  Demux/4 -> Sum3/2
  Demux/5 -> Sum4/2
  Demux/6 -> Sum5/2
  reference/1 -> Demux1/1
  Demux1/1 -> Sum/1
  Demux1/2 -> Sum1/1
  Demux1/3 -> Sum2/1
  Demux1/4 -> Sum3/1
  Demux1/5 -> Sum4/1
  Demux1/6 -> Sum5/1

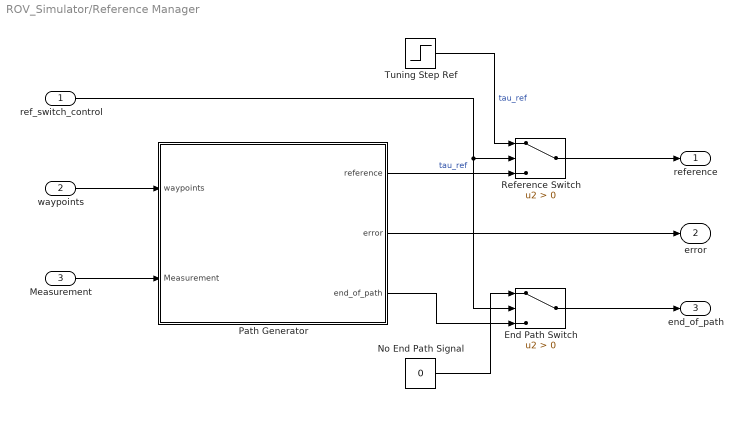
== system ROV_Simulator/Reference Manager ==
  ref_switch_control : Inport
  waypoints : Inport  Port=2
  Measurement : Inport  Port=3
  End Path Switch : Switch  Criteria=u2 > Threshold  SaturateOnIntegerOverflow=off  InputSameDT=off
  No End Path Signal : Constant  Value=0
  Path Generator : Subsystem
  Reference Switch : Switch  Criteria=u2 > Threshold  SaturateOnIntegerOverflow=off  InputSameDT=off
  Tuning Step Ref : Step  Before=[0; 0; 0; 0; 0; 0]  After=step_signal
  reference : Outport
  error : Outport  Port=2
  end_of_path : Outport  Port=3
  wires:
  Measurement/1 -> Path Generator/2(Measurement)
  ref_switch_control/1 -> End Path Switch/2, Reference Switch/2
  Tuning Step Ref/1 -> Reference Switch/1  "tau_ref"
  Reference Switch/1 -> reference/1
  Path Generator/1(reference) -> Reference Switch/3  "tau_ref"
  Path Generator/2(error) -> error/1
  waypoints/1 -> Path Generator/1(waypoints)
  Path Generator/3(end_of_path) -> End Path Switch/3
  End Path Switch/1 -> end_of_path/1
  No End Path Signal/1 -> End Path Switch/1

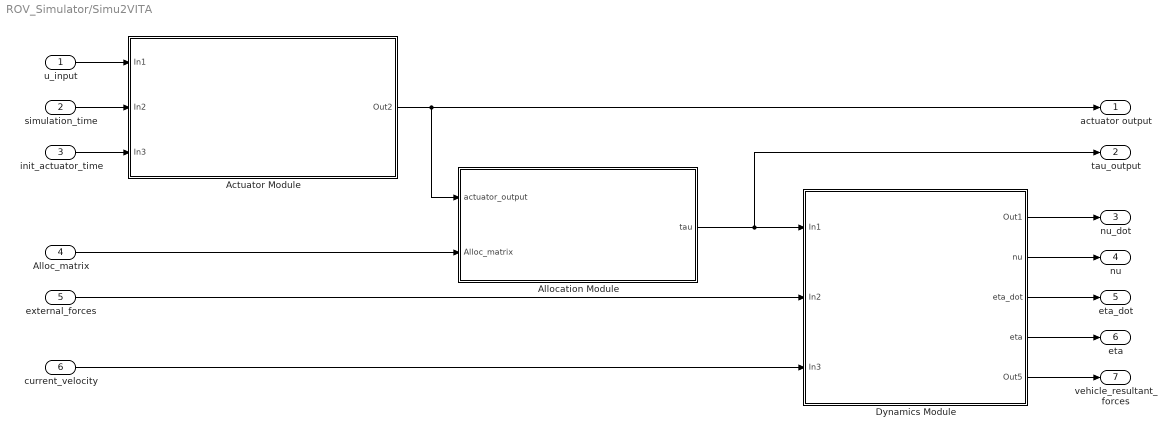
== system ROV_Simulator/Simu2VITA ==
  u_input : Inport
  simulation_time : Inport  Port=2  PortDimensions=1
  init_actuator_time : Inport  Port=3
  Alloc_matrix : Inport  Port=4
  external_forces : Inport  Port=5
  current_velocity : Inport  Port=6
  Actuator Module : Subsystem
  Allocation Module : Subsystem
  Dynamics Module : Subsystem
  actuator output : Outport  VectorParamsAs1DForOutWhenUnconnected=off
  "tau_output " : Outport  Port=2  VectorParamsAs1DForOutWhenUnconnected=off
  nu_dot : Outport  Port=3  VectorParamsAs1DForOutWhenUnconnected=off
  nu : Outport  Port=4  VectorParamsAs1DForOutWhenUnconnected=off
  eta_dot : Outport  Port=5  VectorParamsAs1DForOutWhenUnconnected=off
  eta : Outport  Port=6  VectorParamsAs1DForOutWhenUnconnected=off
  vehicle_resultant_forces : Outport  Port=7
  wires:
  Actuator Module/1(Out2) -> Allocation Module/1(actuator_output), actuator output/1
  u_input/1 -> Actuator Module/1(In1)
  simulation_time/1 -> Actuator Module/2(In2)
  init_actuator_time/1 -> Actuator Module/3(In3)
  Allocation Module/1(tau) -> "tau_output "/1, Dynamics Module/1(In1)
  Alloc_matrix/1 -> Allocation Module/2(Alloc_matrix)
  external_forces/1 -> Dynamics Module/2(In2)
  current_velocity/1 -> Dynamics Module/3(In3)
  Dynamics Module/1(Out1) -> nu_dot/1
  Dynamics Module/2(nu) -> nu/1
  Dynamics Module/3(eta_dot) -> eta_dot/1
  Dynamics Module/4(eta) -> eta/1
  Dynamics Module/5(Out5) -> vehicle_resultant_forces/1

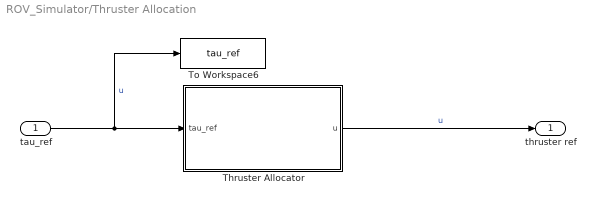
== system ROV_Simulator/Thruster Allocation ==
  tau_ref : Inport
  Thruster Allocator : MATLAB Function  TreatAsAtomicUnit=on
  To Workspace6 : ToWorkspace  VariableName=tau_ref  SaveFormat=Timeseries  SampleTime=-1
      settings: Decimation=6
  thruster ref : Outport  VectorParamsAs1DForOutWhenUnconnected=off
  wires:
  Thruster Allocator/1(u) -> thruster ref/1  "u"
  tau_ref/1 -> Thruster Allocator/1(tau_ref), To Workspace6/1  "u"

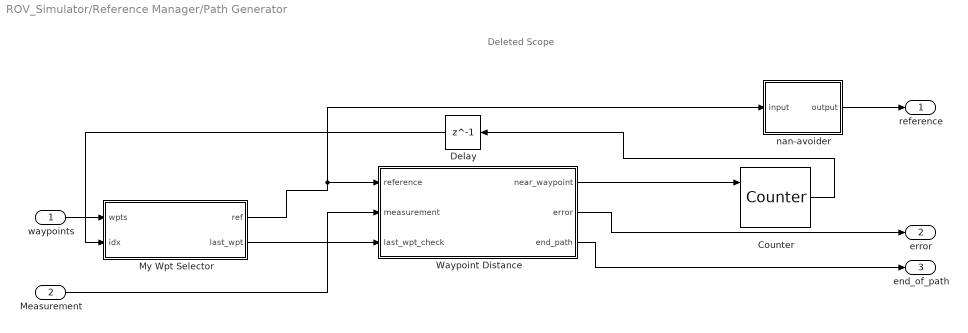
== system ROV_Simulator/Reference Manager/Path Generator ==
  note: Deleted Scope
  waypoints : Inport
  Measurement : Inport  Port=2
  Counter : dspswit3/Counter  Direction=Up  CountEvent=Rising edge  CounterSize=User defined  MaxCount=no_waypoints  InitialCount=1  Output=Count  HitValue=4  ResetInput=on  SamplesPerFrame=1  Ts=1  CntDtype=double  HitDtype=Boolean
  Delay : Delay  DelayLength=1
  My Wpt Selector : MATLAB Function  TreatAsAtomicUnit=on
  "Waypoint Distance " : MATLAB Function  TreatAsAtomicUnit=on
  nan-avoider : MATLAB Function
  reference : Outport  VectorParamsAs1DForOutWhenUnconnected=off
  error : Outport  Port=2  VectorParamsAs1DForOutWhenUnconnected=off
  end_of_path : Outport  Port=3  VectorParamsAs1DForOutWhenUnconnected=off
  wires:
  nan-avoider/1(output) -> reference/1
  My Wpt Selector/1(ref) -> nan-avoider/1(input), "Waypoint Distance "/1(reference)
  "Waypoint Distance "/2(error) -> error/1
  "Waypoint Distance "/1(near_waypoint) -> Counter/1
  Measurement/1 -> "Waypoint Distance "/2(measurement)
  waypoints/1 -> My Wpt Selector/1(wpts)
  Counter/1 -> Delay/1
  Delay/1 -> My Wpt Selector/2(idx)
  "Waypoint Distance "/3(end_path) -> end_of_path/1
  My Wpt Selector/2(last_wpt) -> "Waypoint Distance "/3(last_wpt_check)

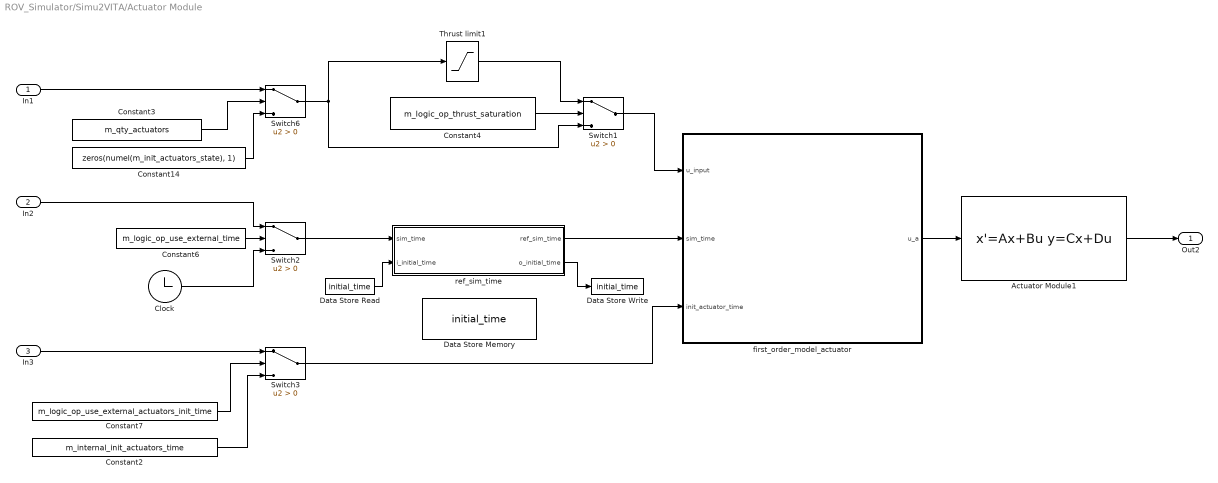
== system ROV_Simulator/Simu2VITA/Actuator Module ==
  In1 : Inport
  In2 : Inport  Port=2
  In3 : Inport  Port=3
  Actuator Module1 : StateSpace  A=m_Ad  B=m_Bd  C=m_Cd  D=m_Dd  InitialCondition=m_init_actuators_state  ContinuousStateAttributes='actuator_state'
  Clock : Clock
  Constant14 : Constant  Value=zeros(numel(m_init_actuators_state), 1)
  Constant2 : Constant  Value=m_internal_init_actuators_time
  Constant3 : Constant  Value=m_qty_actuators
  Constant4 : Constant  Value=m_logic_op_thrust_saturation
  Constant6 : Constant  Value=m_logic_op_use_external_time
  Constant7 : Constant  Value=m_logic_op_use_external_actuators_init_time
  Data Store Memory : DataStoreMemory  DataStoreName=initial_time  ReadBeforeWriteMsg=warning  WriteAfterWriteMsg=warning  WriteAfterReadMsg=warning  InitialValue=-1  ShowAdditionalParam=off
  Data Store Read : DataStoreRead  DataStoreName=initial_time  IndexOptions=Index vector (dialog)  Indices=1  OutputSizes=1
  Data Store Write : DataStoreWrite  DataStoreName=initial_time  IndexOptions=Index vector (dialog)  Indices=1  OutputSizes=1
  Switch{1..3,6} (4 alike) : Switch  Criteria=u2 > Threshold  SaturateOnIntegerOverflow=off  InputSameDT=off
  Thrust limit1 : Saturate  UpperLimit=m_thrust_sup  LowerLimit=m_thrust_inf
  first_order_model_actuator : MATLAB Function  TreatAsAtomicUnit=on
  ref_sim_time : MATLAB Function  TreatAsAtomicUnit=on
  Out2 : Outport
  wires:
  Clock/1 -> Switch2/3
  Constant14/1 -> Switch6/3
  ref_sim_time/2(o_initial_time) -> Data Store Write/1
  Data Store Read/1 -> ref_sim_time/2(i_initial_time)
  Switch6/1 -> Thrust limit1/1, Switch1/3
  In1/1 -> Switch6/1
  Constant2/1 -> Switch3/3
  In2/1 -> Switch2/1
  Switch2/1 -> ref_sim_time/1(sim_time)
  first_order_model_actuator/1(u_a) -> Actuator Module1/1
  Actuator Module1/1 -> Out2/1
  Constant7/1 -> Switch3/2
  Constant3/1 -> Switch6/2
  In3/1 -> Switch3/1
  Constant6/1 -> Switch2/2
  Switch3/1 -> first_order_model_actuator/3(init_actuator_time)
  ref_sim_time/1(ref_sim_time) -> first_order_model_actuator/2(sim_time)
  Constant4/1 -> Switch1/2
  Thrust limit1/1 -> Switch1/1
  Switch1/1 -> first_order_model_actuator/1(u_input)

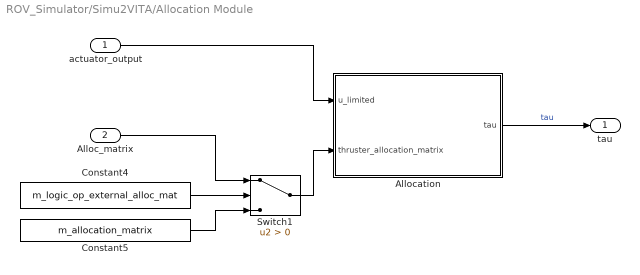
== system ROV_Simulator/Simu2VITA/Allocation Module ==
  actuator_output : Inport
  Alloc_matrix : Inport  Port=2
  Allocation : MATLAB Function  TreatAsAtomicUnit=on
  Constant4 : Constant  Value=m_logic_op_external_alloc_mat
  Constant5 : Constant  Value=m_allocation_matrix
  Switch1 : Switch  Criteria=u2 > Threshold  SaturateOnIntegerOverflow=off  InputSameDT=off
  tau : Outport
  wires:
  Constant5/1 -> Switch1/3
  Constant4/1 -> Switch1/2
  Allocation/1(tau) -> tau/1  "tau"
  Switch1/1 -> Allocation/2(thruster_allocation_matrix)
  actuator_output/1 -> Allocation/1(u_limited)
  Alloc_matrix/1 -> Switch1/1

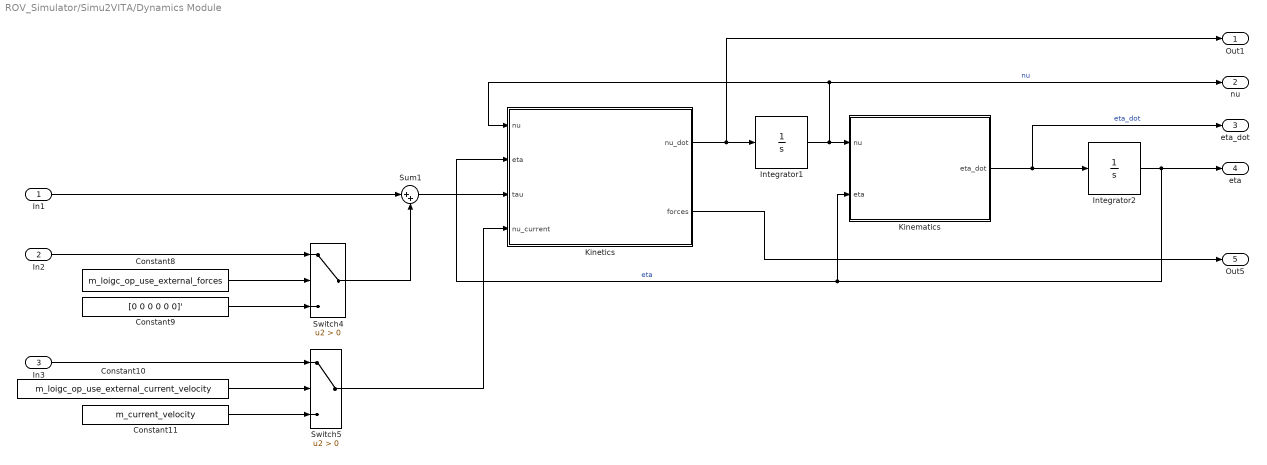
== system ROV_Simulator/Simu2VITA/Dynamics Module ==
  In1 : Inport
  In2 : Inport  Port=2
  In3 : Inport  Port=3
  Constant10 : Constant  Value=m_loigc_op_use_external_current_velocity
  Constant11 : Constant  Value=m_current_velocity
  Constant8 : Constant  Value=m_loigc_op_use_external_forces
  Constant9 : Constant  Value=[0 0 0 0 0 0]'
  Integrator1 : Integrator  InitialCondition=m_nu_0
  Integrator2 : Integrator  InitialCondition=m_eta_0
  Kinematics : MATLAB Function  TreatAsAtomicUnit=on
  Kinetics : Subsystem
  Sum1 : Sum  Inputs=|++
  Switch4 : Switch  Criteria=u2 > Threshold  SaturateOnIntegerOverflow=off  InputSameDT=off
  Switch5 : Switch  Criteria=u2 > Threshold  SaturateOnIntegerOverflow=off  InputSameDT=off
  Out1 : Outport
  nu : Outport  Port=2
  eta_dot : Outport  Port=3
  eta : Outport  Port=4
  Out5 : Outport  Port=5
  wires:
  Kinetics/2(forces) -> Out5/1
  In1/1 -> Sum1/1
  Constant10/1 -> Switch5/2
  Constant11/1 -> Switch5/3
  In2/1 -> Switch4/1
  Kinetics/1(nu_dot) -> Out1/1, Integrator1/1
  Sum1/1 -> Kinetics/3(tau)
  In3/1 -> Switch5/1
  Integrator1/1 -> Kinematics/1(nu), Kinetics/1(nu), nu/1  "nu"
  Switch5/1 -> Kinetics/4(nu_current)
  Kinematics/1(eta_dot) -> eta_dot/1, Integrator2/1  "eta_dot"
  Constant8/1 -> Switch4/2
  Integrator2/1 -> Kinetics/2(eta), Kinematics/2(eta), eta/1  "eta"
  Switch4/1 -> Sum1/2
  Constant9/1 -> Switch4/3

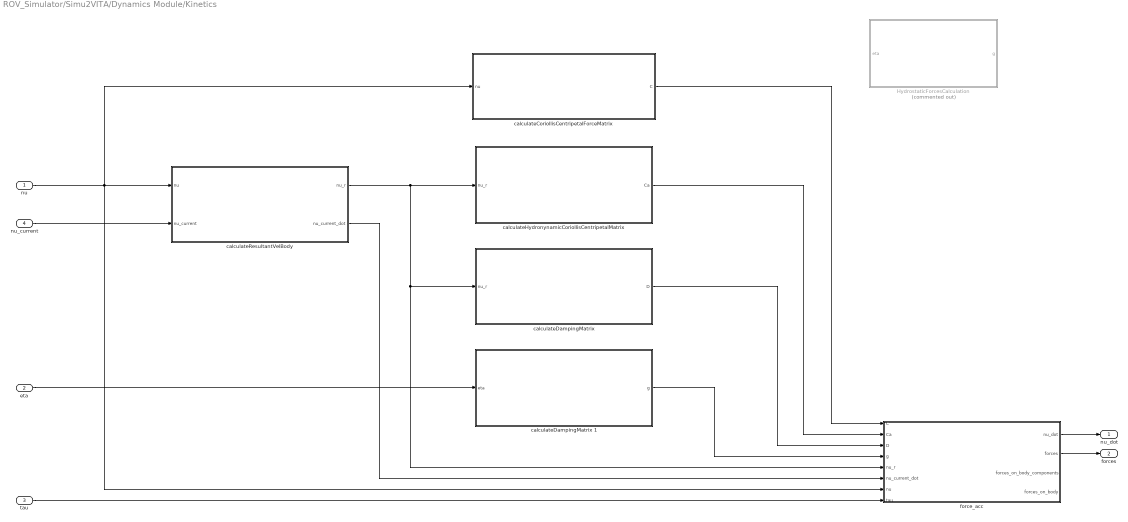
== system ROV_Simulator/Simu2VITA/Dynamics Module/Kinetics ==
  nu : Inport
  eta : Inport  Port=2
  tau : Inport  Port=3
  nu_current : Inport  Port=4
  HydrostaticForcesCalculation : Subsystem  Commented=on
  calculateCoriollisCentripetalForceMatrix : MATLAB Function  TreatAsAtomicUnit=on
  "calculateDampingMatrix " : MATLAB Function  TreatAsAtomicUnit=on
  calculateDampingMatrix 1 : MATLAB Function  TreatAsAtomicUnit=on
  calculateHydronynamicCoriollisCentripetalMatrix : MATLAB Function  TreatAsAtomicUnit=on
  calculateResultantVelBody : MATLAB Function  TreatAsAtomicUnit=on
  force_acc : MATLAB Function  TreatAsAtomicUnit=on
  nu_dot : Outport
  forces : Outport  Port=2
  wires:
  calculateCoriollisCentripetalForceMatrix/1(C) -> force_acc/1(C)
  nu/1 -> force_acc/7(nu), calculateCoriollisCentripetalForceMatrix/1(nu), calculateResultantVelBody/1(nu)
  calculateResultantVelBody/1(nu_r) -> force_acc/5(nu_r), "calculateDampingMatrix "/1(nu_r), calculateHydronynamicCoriollisCentripetalMatrix/1(nu_r)
  force_acc/2(forces) -> forces/1
  force_acc/1(nu_dot) -> nu_dot/1
  nu_current/1 -> calculateResultantVelBody/2(nu_current)
  calculateResultantVelBody/2(nu_current_dot) -> force_acc/6(nu_current_dot)
  tau/1 -> force_acc/8(tau)
  calculateHydronynamicCoriollisCentripetalMatrix/1(Ca) -> force_acc/2(Ca)
  "calculateDampingMatrix "/1(D) -> force_acc/3(D)
  eta/1 -> calculateDampingMatrix 1/1(eta)
  calculateDampingMatrix 1/1(g) -> force_acc/4(g)

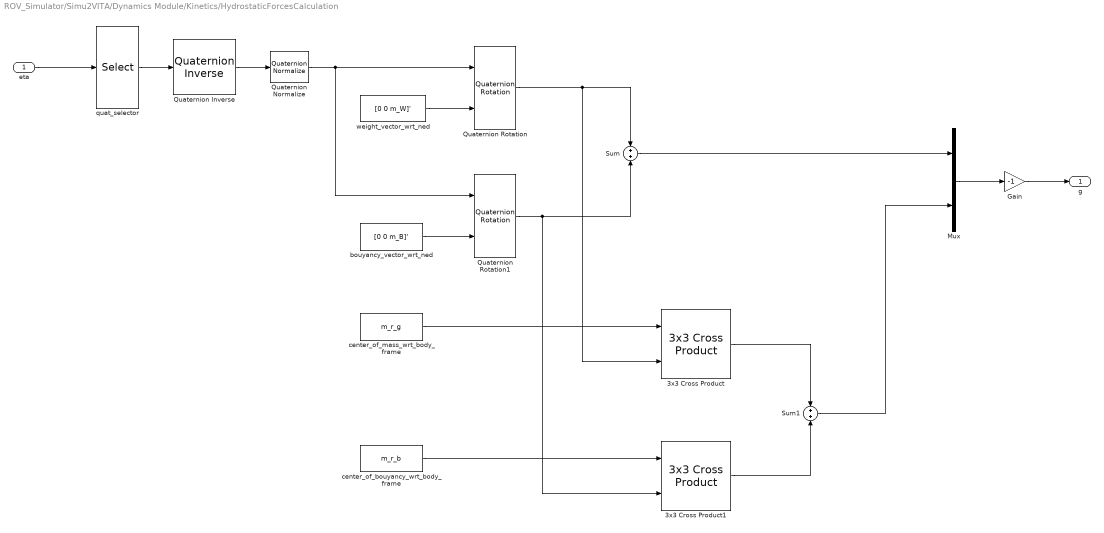
== system ROV_Simulator/Simu2VITA/Dynamics Module/Kinetics/HydrostaticForcesCalculation ==
  eta : Inport
  3x3 Cross Product : sharedutil/3x3 Cross Product  aMode=aMode
  3x3 Cross Product1 : sharedutil/3x3 Cross Product  aMode=aMode
  Gain : Gain  Gain=-1
  Mux : Mux  Inputs=2
  Quaternion Inverse : aerolibutil/Quaternion Inverse
  Quaternion Normalize : sharedutil/Quaternion Normalize  aMode=aMode
  Quaternion Rotation : aerolibutil/Quaternion Rotation
  Quaternion Rotation1 : aerolibutil/Quaternion Rotation
  Sum : Sum  Inputs=+|+
  Sum1 : Sum  Inputs=+|+
  bouyancy_vector_wrt_ned : Constant  Value=[0 0 m_B]'
  center_of_bouyancy_wrt_body_frame : Constant  Value=m_r_b
  center_of_mass_wrt_body_frame : Constant  Value=m_r_g
  quat_selector : Selector  InputPortWidth=7  IndexOptions=Index vector (dialog)  Indices=[4 5 6 7]  OutputSizes=1
  weight_vector_wrt_ned : Constant  Value=[0 0 m_W]'
  g : Outport
  wires:
  eta/1 -> quat_selector/1
  quat_selector/1 -> Quaternion Inverse/1
  weight_vector_wrt_ned/1 -> Quaternion Rotation/2
  bouyancy_vector_wrt_ned/1 -> Quaternion Rotation1/2
  Quaternion Rotation/1 -> 3x3 Cross Product/2, Sum/1
  Sum/1 -> Mux/1
  Mux/1 -> Gain/1
  Quaternion Rotation1/1 -> 3x3 Cross Product1/2, Sum/2
  center_of_mass_wrt_body_frame/1 -> 3x3 Cross Product/1
  center_of_bouyancy_wrt_body_frame/1 -> 3x3 Cross Product1/1
  3x3 Cross Product/1 -> Sum1/1
  3x3 Cross Product1/1 -> Sum1/2
  Sum1/1 -> Mux/2
  Gain/1 -> g/1
  Quaternion Inverse/1 -> Quaternion Normalize/1
  Quaternion Normalize/1 -> Quaternion Rotation1/1, Quaternion Rotation/1

== matlab function ROV_Simulator/Simu2VITA/Dynamics Module/Kinetics/calculateDampingMatrix  ==
  data: D output; nu_r input; m_Dlf parameter; m_Dqf parameter
function D = calculateDampingMatrix(nu_r, m_Dlf, m_Dqf)
            
    [velRow, velCols] = size(nu_r);

    if(velRow == 1 || velCols ~= 1)
        
        ME = MException('MyComponent:incompatiblePosition', ...
                'Position vector does not match a column vector!');

        throw(ME);
        
    else

        tmpMtrx = abs([nu_r nu_r nu_r nu_r nu_r nu_r]);

        D = m_Dlf + m_Dqf.*tmpMtrx;

    end

end
